simulink model "UnifiedPowerFlowController"  (R2024a)
settings: Solver=FixedStepDiscrete  StartTime=0.0  StopTime=0.8  FixedStep=Ts  RelTol=1e-3
PreLoadFcn:
  | Ts=1/512/60;
undefined symbols (not defined in the file or in its folder): DiscIntNeverNeededParam
libraries: spsabctodq0Lib x10, spsMeanVariableFrequencyLib x10, spsThreeLevelBridgeLib x8, spsVoltageMeasurementLib x8, spsZigzagPhaseShiftingTransformerLib x8, spsCurrentMeasurementLib x6, spsSecondOrderFilterLib x5, spsThreePhaseVIMeasurementLib x4, spsSeriesRLCBranchLib x4, spsDistributedParametersLineLib x3, spsPowerPositiveSequenceLib x3, spsThreePhaseSourceLib x2
(part 1 of 7)
settings Model: Creator=The MathWorks, Inc.  LastModifiedBy=Monia
settings SolverCC: AlgebraicLoopSolver=TrustRegion
settings DataIOCC: InitialState=xInitial_upfc  SaveFinalState=on  SaveFormat=Structure  SaveOutput=off  SaveTime=off  ReturnWorkspaceOutputs=off  SignalLoggingName=sigsOut
settings OptimizationCC: BlockReduction=off  BooleanDataType=off  ExpressionDepthLimit=2147483647  InitFltsAndDblsToZero=on  EfficientMapNaN2IntZero=off  LifeSpan=inf
settings DebuggingCC: UnderspecifiedInitializationDetection=Classic  MergeDetectMultiDrivingBlocksExec=none  SignalResolutionControl=TryResolveAllWithWarning  MultiTaskDSMMsg=warning  MultiTaskCondExecSysMsg=none  FcnCallInpInsideContextMsg=warning  UnconnectedInputMsg=warning  UnconnectedOutputMsg=warning  UnconnectedLineMsg=warning  StateNameClashWarn=warning  SFUnexpectedBacktrackingDiag=warning  SFNoUnconditionalDefaultTransitionDiag=warning  SFExecutionAtInitializationDiag=none  ArithmeticOperatorsInVariantConditions=warning
settings HardwareCC: ProdBitPerPointer=32  ProdBitPerSizeT=32  ProdBitPerPtrDiffT=32  ProdLargestAtomicFloat=None  ProdIntDivRoundTo=Undefined  ProdEndianess=Unspecified  ProdWordSize=32  ProdHWDeviceType=32-bit Generic  TargetBitPerPointer=64  TargetBitPerSizeT=64  TargetBitPerPtrDiffT=64  TargetLongLongMode=on  TargetIntDivRoundTo=Zero  TargetEndianess=LittleEndian  TargetWordSize=64  TargetHWDeviceType=MATLAB Host  ProdEqTarget=off
settings ModelReferenceCC: EnableRefExpFcnMdlSchedulingChecks=on  PropagateSignalLabelsOutOfModel=off
settings SFSimCC: SimUseLocalCustomCode=off  CustomCodeUndefinedFunction=UseInterfaceOnly
settings RTWCC: SystemTargetFile=accel.tlc  TemplateMakefile=accel_default_tmf  RTWUseLocalCustomCode=off  GPUComputeCapability=3.5  DLArmComputeVersion=19.05
settings CodeAppCC: StateflowObjectComments=on
settings STFCustomTargetCC: TargetLangStandard=C89/C90 (ANSI)  MATLABClassNameForMDSCustomization=Simulink.SoftwareTarget.TargetSpecificTriggerConfigurationBase  UseToolchainInfoCompliant=off  SystemTargetFile=accel.tlc
settings ConfigComp: CovMetricSettings=dw  CovSaveCumulativeToWorkspaceVar=on  CovSaveSingleToWorkspaceVar=on  CovExternalEMLEnable=off  CovSFcnEnable=off
settings SimscapeCC: SimscapeNormalizeSystem=off

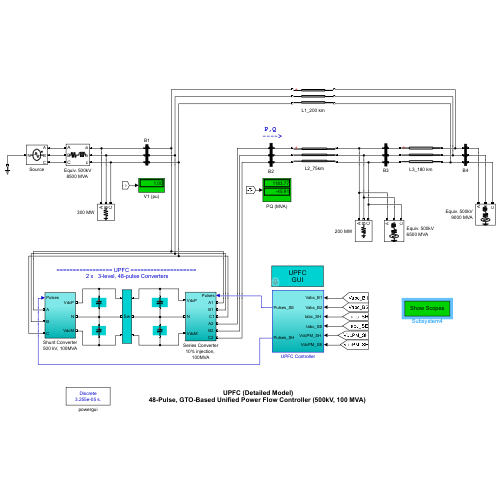
[thumbnail: Simulink's stored preview of the top-level diagram]
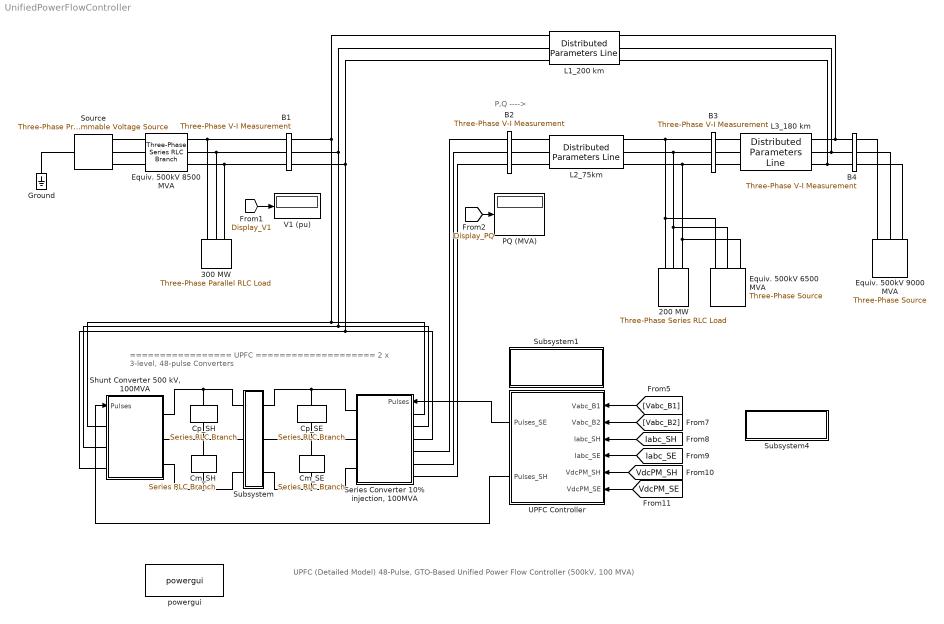
== system UnifiedPowerFlowController ==
  note: ================= UPFC ====================
      | 2 x   3-level, 48-pulse Converters
  note: P,Q
      | ---->
  note: UPFC (Detailed Model)
      | 48-Pulse, GTO-Based Unified Power Flow Controller (500kV, 100 MVA)
  200 MW : spsThreePhaseSeriesRLCLoadLib/Three-Phase Series RLC Load  LConnTagsString=A|B|C  Configuration=Y (grounded)  NominalVoltage=500e3  Vabc=[1e3 1e3 1e3]  Vabcp=[1e3 1e3 1e3]  NominalFrequency=60  UnbalancedPower=off  ActivePower=200e6  InductivePower=0  CapacitivePower=0  Pabc=[10e3 9e3 11e3]  QLabc=[100 90 110]  QCabc=[100 90 110]  Pabcp=[10e3 9e3 11e3]  QLabcp=[100 90 110]  QCabcp=[100 90 110]  Measurements=None  LoadType=constant Z
  300 MW : spsThreePhaseParallelRLCLoadLib/Three-Phase Parallel RLC Load  LConnTagsString=A|B|C  Configuration=Y (grounded)  NominalVoltage=500e3  Vabc=[1e3 1e3 1e3]  Vabcp=[1e3 1e3 1e3]  NominalFrequency=60  UnbalancedPower=off  ActivePower=300e6  InductivePower=0  CapacitivePower=0  Pabc=[10e3 9e3 11e3]  QLabc=[100 90 110]  QCabc=[100 90 110]  Pabcp=[10e3 9e3 11e3]  QLabcp=[100 90 110]  QCabcp=[100 90 110]  Measurements=None  LoadType=constant Z
  B1 : spsThreePhaseVIMeasurementLib/Three-Phase V-I Measurement  VoltageMeasurement=phase-to-ground  SetLabelV=on  LabelV=Vabc_B1  Vpu=on  VpuLL=off  CurrentMeasurement=yes  SetLabelI=on  LabelI=Iabc_B1  Ipu=on  Pbase=100e6  Vbase=500e3  OutputType=Magnitude  PhasorSimulation=off  PSBequivalent=0
  B2 : spsThreePhaseVIMeasurementLib/Three-Phase V-I Measurement  VoltageMeasurement=phase-to-ground  SetLabelV=on  LabelV=Vabc_B2  Vpu=on  VpuLL=off  CurrentMeasurement=yes  SetLabelI=on  LabelI=Iabc_B2  Ipu=on  Pbase=100e6  Vbase=500e3  OutputType=Magnitude  PhasorSimulation=off  PSBequivalent=0
  B3 : spsThreePhaseVIMeasurementLib/Three-Phase V-I Measurement  VoltageMeasurement=phase-to-ground  SetLabelV=on  LabelV=Vabc_B3  Vpu=on  VpuLL=off  CurrentMeasurement=yes  SetLabelI=on  LabelI=Iabc_B3  Ipu=on  Pbase=100e6  Vbase=500e3  OutputType=Magnitude  PhasorSimulation=off  PSBequivalent=0
  B4 : spsThreePhaseVIMeasurementLib/Three-Phase V-I Measurement  VoltageMeasurement=phase-to-ground  SetLabelV=on  LabelV=Vabc_B4  Vpu=on  VpuLL=off  CurrentMeasurement=no  SetLabelI=on  LabelI=Iabc_B4  Ipu=on  Pbase=100e6  Vbase=500e3  OutputType=Magnitude  PhasorSimulation=off  PSBequivalent=0
  Cm_SE : spsSeriesRLCBranchLib/Series RLC Branch  LConnTagsString=__new0  RConnTagsString=__new0  BranchType=C  Resistance=1.0  Inductance=1.0  SetiL0=off  InitialCurrent=0  Capacitance=2500e-6  Setx0=off  InitialVoltage=0  Measurements=Branch voltage
  Cm_SH : spsSeriesRLCBranchLib/Series RLC Branch  LConnTagsString=__new0  RConnTagsString=__new0  BranchType=C  Resistance=1.0  Inductance=1.0  SetiL0=off  InitialCurrent=0  Capacitance=2500e-6  Setx0=off  InitialVoltage=0  Measurements=Branch voltage
  Cp_SE : spsSeriesRLCBranchLib/Series RLC Branch  LConnTagsString=__new0  RConnTagsString=__new0  BranchType=C  Resistance=1.0  Inductance=1.0  SetiL0=off  InitialCurrent=0  Capacitance=2500e-6  Setx0=off  InitialVoltage=0  Measurements=Branch voltage
  Cp_SH : spsSeriesRLCBranchLib/Series RLC Branch  LConnTagsString=__new0  RConnTagsString=__new0  BranchType=C  Resistance=1.0  Inductance=1.0  SetiL0=off  InitialCurrent=0  Capacitance=2500e-6  Setx0=off  InitialVoltage=0  Measurements=Branch voltage
  Equiv. 500kV 6500 MVA : spsThreePhaseSourceLib/Three-Phase Source  InternalConnection=Yg  VoltagePhases=off  Voltage=500e3*1.00  PhaseAngle=9.2-20  Voltage_phases=[25e3 25e3 25e3]/sqrt(3)  PhaseAngles_phases=[0 -120 +120]  Frequency=60  NonIdealSource=on  SpecifyImpedance=on  Resistance=0.8929  Inductance=16.58e-3  ShortCircuitLevel=6500e6  BaseVoltage=500e3  XRratio=8  BusType=swing  Pref=0  Qref=0  Prefabc=[10e3, 10e3, 10e3]  Qrefabc=[0, 0, 0]  Qmin=-inf  Qmax=inf
  "Equiv. 500kV 8500 MVA " : spsThreePhaseSeriesRLCBranchLib/Three-Phase Series RLC Branch  LConnTagsString=A|B|C  RConnTagsString=A|B|C  BranchType=RL  Resistance=500e3^2/8500e6/10  Inductance=500e3^2/8500e6/(2*pi*60)  Capacitance=1.0  Measurements=None
  Equiv. 500kV 9000 MVA : spsThreePhaseSourceLib/Three-Phase Source  InternalConnection=Yg  VoltagePhases=off  Voltage=500e3*0.98  PhaseAngle=9.2-40  Voltage_phases=[25e3 25e3 25e3]/sqrt(3)  PhaseAngles_phases=[0 -120 +120]  Frequency=60  NonIdealSource=on  SpecifyImpedance=on  Resistance=0.8929  Inductance=16.58e-3  ShortCircuitLevel=9000e6  BaseVoltage=500e3  XRratio=10  BusType=swing  Pref=0  Qref=0  Prefabc=[10e3, 10e3, 10e3]  Qrefabc=[0, 0, 0]  Qmin=-inf  Qmax=inf
  Ground : spsGroundLib/Ground  LConnTagsString=a
  L1_200 km : spsDistributedParametersLineLib/Distributed Parameters Line  Phases=3  Length=200  Frequency=60  Resistance=[0.01273*2 0.3864]  Inductance="[0.9337e-3  4.1264e-3]"  Capacitance=[12.74e-9 7.751e-9]  x1=[-0.00113932291666667 -1.30080473974736e-10 4414.79498015263 -499890.552538387;-0.00110677083333333 -1.3001617192128e-10 10548.8886083546 -499798.73537353;-0.00107421875 -1.2993228991057e-10 16681.393612734 -499631.650357529;-0.00104166666666667 -1.29828840574929e-10 22811.3864605943 -499389.322652774;-0.00100911458333333 -1.29705839493444e-10 28937.9439975605 -499071.788752926;-0.0009765625 -1.29563305189627e-10 35060.1435866028 -498679.096477422;-0.000944010416666667 -1.2940125912862e-10 41177.0632469823 -498211.304964274;-0.000911458333333333 -1.29219725713964e-10 47287.7817930979 -497668.484661164;-0.00087890625 -1.29018732283922e-10 53391.3789732137 -497050.717314833;-0.000846354166666667 -1.28798309107367e-10 59486.935608045 -496358.09595877;-0.000813802083333333 -1.28558489379218e-10 65573.5337291838 -495590.724899204;-0.00078125 -1.28299309215443e-10 71650.2567173415 -494748.719699394;-0.000748697916666667 -1.28020807647623e-10 77716.1894403879 -493832.207162227;-0.000716145833333333 -1.27723026617068e-10 83770.4183911672 -492841.325311118;-0.00068359375 -1.27406010968507e-10 89812.0318250686 -491776.223369231;-0.000651041666666667 -1.2706980844333e-10 95840.1198973318 -490637.061736999;-0.000618489583333333 -1.26714469672401e-10 101853.774800066 -489424.011967975;-0.0005859375 -1.26340048168432e-10 107852.090898963 -488137.256742991;-0.000553385416666667 -1.25946600317924e-10 113834.164869682 -486776.989842652;-0.000520833333333333 -1.25534185372677e-10 119799.095833886 -485343.416118148;-0.00048828125 -1.25102865440863e-10 125745.985494914 -483836.751460411;-0.000455729166666667 -1.24652705477678e-10 131673.938273056 -482257.222767596;-0.000423177083333333 -1.24183773275557e-10 137582.061440429 -480605.067910913;-0.000390625 -1.23696139453964e-10 143469.465255415 -478880.535698807;-0.000358072916666667 -1.2318987744876e-10 149335.263096657 -477083.885839486;-0.000325520833333333 -1.2266506350114e-10 155178.571596574 -475215.388901809;-0.00029296875 -1.22121776646154e-10 160998.5107744 -473275.326274544;-0.000260416666666667 -1.21560098700805e-10 166794.204168703 -471263.990123985;-0.000227864583333333 -1.20980114251724e-10 172564.778969376 -469181.683349959;-0.0001953125 -1.20381910642437e-10 178309.366149078 -467028.719540206;-0.000162760416666667 -1.19765577960207e-10 184027.100594112 -464805.422923158;-0.000130208333333333 -1.19131209022468e-10 189717.121234702 -462512.128319105;-9.765625e-05 -1.1847889936285e-10 195378.571174668 -460149.181089781;-6.51041666666667e-05 -1.17808747216787e-10 201010.597820474 -457716.937086347;-3.25520833333333e-05 -1.17120853506728e-10 206612.353009623 -455215.762595802]  x2=[-0.00113932291666667 -1.05841083346228e-10 -126400.807658291 -476001.468702008;-0.00110677083333333 -1.0642802292755e-10 -120550.019662708 -477516.759017374;-0.00107421875 -1.06998934840092e-10 -114681.077277581 -478960.137065278;-0.00104166666666667 -1.0755373310662e-10 -108794.864344047 -480331.385478293;-0.00100911458333333 -1.08092334176555e-10 -102892.267304122 -481630.297751453;-0.0009765625 -1.08614656938559e-10 -96974.175067208 -482856.678273347;-0.000944010416666667 -1.09120622732743e-10 -91041.4788762281 -484010.34235558;-0.000911458333333333 -1.09610155362522e-10 -85095.0721734062 -485091.116260584;-0.00087890625 -1.1008318110608e-10 -79135.8504657194 -486098.837227784;-0.000846354166666667 -1.10539628727482e-10 -73164.7111900368 -487033.35349811;-0.000813802083333333 -1.10979429487394e-10 -67182.5535779701 -487894.524336849;-0.00078125 -1.1140251715344e-10 -61190.2785204513 -488682.220054839;-0.000748697916666667 -1.11808828010173e-10 -55188.7884320629 -489396.322028004;-0.000716145833333333 -1.12198300868673e-10 -49178.987115137 -490036.722715212;-0.00068359375 -1.1257087707576e-10 -43161.7796236461 -490603.325674476;-0.000651041666666667 -1.12926500522828e-10 -37138.0721269053 -491096.045577475;-0.000618489583333333 -1.13265117654293e-10 -31108.7717731068 -491514.808222403;-0.0005859375 -1.13586677475661e-10 -25074.7865527063 -491859.550545146;-0.000553385416666667 -1.13891131561206e-10 -19037.0251616833 -492130.220628778;-0.000520833333333333 -1.14178434061263e-10 -12996.3968646946 -492326.777711381;-0.00048828125 -1.14448541709131e-10 -6953.8113581426 -492449.192192181;-0.000455729166666667 -1.14701413827592e-10 -910.178633178191 -492497.445636008;-0.000423177083333333 -1.14937012335036e-10 5133.59116134048 -492471.530776069;-0.000390625 -1.15155301751194e-10 11176.5878559131 -492371.451515048;-0.000358072916666667 -1.15356249202483e-10 17217.9013974653 -492197.222924514;-0.000325520833333333 -1.15539824426955e-10 23256.6219863995 -491948.871242651;-0.00029296875 -1.15705999778858e-10 29291.8402136071 -491626.433870309;-0.000260416666666667 -1.15854750232794e-10 35322.6471974224 -491229.95936537;-0.000227864583333333 -1.15986053387492e-10 41348.1347204966 -490759.507435436;-0.0001953125 -1.16099889469181e-10 47367.3953665724 -490215.148928839;-0.000162760416666667 -1.16196241334564e-10 53379.5226571369 -489596.965823965;-0.000130208333333333 -1.16275094473405e-10 59383.6111879346 -488905.051216918;-9.765625e-05 -1.16336437010713e-10 65378.7567653174 -488139.509307491;-6.51041666666667e-05 -1.16380259708525e-10 71364.0565424134 -487300.455383481;-3.25520833333333e-05 -1.16406555967306e-10 77338.6091550917 -486388.015803322]  x3=[-0.00113932291666667 -2.8339490666223e-13 -16.9421274649165 53.6415754395801;-0.00110677083333333 -2.86603709471157e-13 -17.5991164005906 53.4296303617768;-0.00107421875 -2.89769350815649e-13 -18.2534549740693 53.2096389781707;-0.00104166666666667 -2.92891353961764e-13 -18.9050446443705 52.9816344186548;-0.00100911458333333 -2.95969248747311e-13 -19.5537872844865 52.7456510198773;-0.0009765625 -2.99002571652657e-13 -20.1995851961618 52.50172432007;-0.000944010416666667 -3.0199086587053e-13 -20.8423411246066 52.2498910536966;-0.000911458333333333 -3.04933681374813e-13 -21.4819582731421 51.9901891459206;-0.00087890625 -3.07830574988315e-13 -22.1183403177786 51.7226577068943;-0.000846354166666667 -3.10681110449514e-13 -22.7513914217208 51.4473370258682;-0.000813802083333333 -3.13484858478254e-13 -23.3810162498012 51.1642685651241;-0.00078125 -3.16241396840395e-13 -24.0071199828364 50.8734949537312;-0.000748697916666667 -3.18950310411399e-13 -24.6296083319074 50.5750599811256;-0.000716145833333333 -3.21611191238846e-13 -25.2483875525584 50.2690085905165;-0.00068359375 -3.24223638603872e-13 -25.8633644589148 49.9553868721177;-0.000651041666666667 -3.26787259081513e-13 -26.4744464377167 49.6342420562063;-0.000618489583333333 -3.29301666599954e-13 -27.0815414622657 49.3056225060103;-0.0005859375 -3.31766482498671e-13 -27.6845581062843 48.9695777104252;-0.000553385416666667 -3.34181335585458e-13 -28.2834055576838 48.6261582765612;-0.000520833333333333 -3.3654586219232e-13 -28.8779936322409 48.2754159221218;-0.00048828125 -3.3885970623025e-13 -29.4682327871786 47.9174034676155;-0.000455729166666667 -3.41122519242845e-13 -30.0540341346512 47.552174828401;-0.000423177083333333 -3.43333960458789e-13 -30.6353094551306 47.179785006568;-0.000390625 -3.4549369684317e-13 -31.2119712106915 46.800290082654;-0.000358072916666667 -3.47601403147632e-13 -31.7839325581948 46.4137472071984;-0.000325520833333333 -3.49656761959359e-13 -32.3511073623653 46.0202145921366;-0.00029296875 -3.51659463748873e-13 -32.9134102087637 45.619751502033;-0.000260416666666667 -3.53609206916652e-13 -33.4707564166498 45.2124182451557;-0.000227864583333333 -3.55505697838545e-13 -34.0230620517346 44.7982761643951;-0.0001953125 -3.57348650909997e-13 -34.5702439388211 44.3773876280251;-0.000162760416666667 -3.59137788589054e-13 -35.1122196743297 43.9498160203112;-0.000130208333333333 -3.60872841438162e-13 -35.6489076387083 43.5156257319647;-9.765625e-05 -3.62553548164744e-13 -36.1802270087235 43.0748821504461;-6.51041666666667e-05 -3.64179655660549e-13 -36.7060977696325 42.6276516501175;-3.25520833333333e-05 -3.65750919039769e-13 -37.226440727233 42.1740015822472]  x4=[-0.00113932291666667 -5.53609918313425e-14 -894.269601115783 -3549.34214309645;-0.00110677083333333 -6.65829424292671e-14 -850.646376261383 -3560.04894780867;-0.00107421875 -7.77948658809732e-14 -806.895047191641 -3570.21962224425;-0.00104166666666667 -8.89950737120296e-14 -763.022202695785 -3579.85263473701;-0.00100911458333333 -1.00181879212335e-13 -719.034449862819 -3588.94653459072;-0.0009765625 -1.11353597690128e-13 -674.938413086521 -3597.4999522975;-0.000944010416666667 -1.225085467257e-13 -630.740733067831 -3605.51159974411;-0.000911458333333333 -1.33645046424757e-13 -586.448065814787 -3612.98027040591;-0.00087890625 -1.44761419671408e-13 -542.067081640157 -3619.90483952857;-0.000846354166666667 -1.5585599238073e-13 -497.604464156912 -3626.28426429746;-0.000813802083333333 -1.66927093750883e-13 -453.066909271697 -3632.11758399467;-0.00078125 -1.77973056514724e-13 -408.461124176457 -3637.4039201437;-0.000748697916666667 -1.8899221719089e-13 -363.793826338355 -3642.14247664178;-0.000716145833333333 -1.99982916334315e-13 -319.071742488145 -3646.33253987974;-0.00068359375 -2.10943498786134e-13 -274.301607607154 -3649.97347884945;-0.000651041666666667 -2.21872313922948e-13 -229.490163913017 -3653.06474523891;-0.000618489583333333 -2.32767715905396e-13 -184.644159844327 -3655.60587351476;-0.0005859375 -2.43628063926015e-13 -139.770349044339 -3657.59648099244;-0.000553385416666667 -2.54451722456341e-13 -94.8754893439008 -3659.03626789378;-0.000520833333333333 -2.65237061493213e-13 -49.9663417437466 -3659.92501739216;-0.00048828125 -2.75982456804242e-13 -5.04966939631674 -3660.26259564519;-0.000455729166666667 -2.86686290172419e-13 39.8677634127503 -3660.04895181481;-0.000423177083333333 -2.97346949639812e-13 84.7791922832927 -3659.28411807502;-0.000390625 -3.07962829750317e-13 129.677853719319 -3657.96820960694;-0.000358072916666667 -3.18532331791438e-13 174.556986147569 -3656.10142458156;-0.000325520833333333 -3.29053864035045e-13 219.409830935775 -3653.68404412984;-0.00029296875 -3.39525841977084e-13 264.229633410495 -3650.71643230038;-0.000260416666666667 -3.49946688576195e-13 309.009643874337 -3647.1990360046;-0.000227864583333333 -3.60314834491212e-13 353.743118622438 -3643.13238494946;-0.0001953125 -3.70628718317496e-13 398.423320958044 -3638.51709155763;-0.000162760416666667 -3.80886786822081e-13 443.043522207029 -3633.35385087534;-0.000130208333333333 -3.91087495177583e-13 487.597002731213 -3627.64344046763;-9.765625e-05 -4.01229307194844e-13 532.077052940308 -3621.3867203013;-6.51041666666667e-05 -4.11310695554278e-13 576.476974302363 -3614.58463261541;-3.25520833333333e-05 -4.21330142035882e-13 620.790080352538 -3607.23820177933]  x5=0.00113108313399148  V1=ones(3,3)  V2=ones(3,3)  I1=ones(3,3)  I2=ones(3,3)  nHarmo=1  Measurements=None  Decoupling=off  VsMag0=0  VrMag0=0  VsAngle0=0  VrAngle0=0  IsMag0=0  IrMag0=0  IsAngle0=0  IrAngle0=0
      settings: AttributesFormatString=\n
  L2_75km : spsDistributedParametersLineLib/Distributed Parameters Line  Phases=3  Length=75  Frequency=60  Resistance=[0.01273*2 0.3864]  Inductance="[0.9337e-3  4.1264e-3]"  Capacitance=[12.74e-9 7.751e-9]  x1=[-0.000455729166666667 -2.0819094293585e-10 0 0;-0.000423177083333333 -2.08074842291704e-10 0 0;-0.000390625 -2.07927406341667e-10 0 0;-0.000358072916666667 -2.07748657289053e-10 0 0;-0.000325520833333333 -2.0753862205281e-10 0 0;-0.00029296875 -2.07297332263474e-10 0 0;-0.000260416666666667 -2.07024824258398e-10 166794.132131736 -471263.82102114;-0.000227864583333333 -2.06721139076285e-10 172564.704862681 -469181.515143851;-0.0001953125 -2.06386322451008e-10 178309.289983816 -467028.552256167;-0.000162760416666667 -2.06020424804719e-10 184027.022381753 -464805.256586379;-0.000130208333333333 -2.05623501240256e-10 189717.040987023 -462511.962954637;-9.765625e-05 -2.0519561153285e-10 195378.488903755 -460149.016722528;-6.51041666666667e-05 -2.04736820121115e-10 201010.513538717 -457716.77374106;-3.25520833333333e-05 -2.04247196097352e-10 206612.266729715 -455215.600297082]  x2=[-0.000455729166666667 1.24391145626069e-11 0 0;-0.000423177083333333 1.15584511756505e-11 0 0;-0.000390625 1.06760471284624e-11 0 0;-0.000358072916666667 9.79203530784625e-12 0 0;-0.000325520833333333 8.90654884273071e-12 0 0;-0.00029296875 8.01972108412033e-12 0 0;-0.000260416666666667 7.13168558501352e-12 120220.444766576 -484737.668130302;-0.000227864583333333 6.24257608029001e-12 126159.86924118 -483225.878484715;-0.0001953125 5.35252646657081e-12 132080.294503528 -481641.316799273;-0.000162760416666667 4.46167078205388e-12 137980.828959354 -479984.221703137;-0.000130208333333333 3.5701431863285e-12 143860.584009871 -478254.842748733;-9.765625e-05 2.67807794017127e-12 149718.674185598 -476453.440374171;-6.51041666666667e-05 1.78560938532699e-12 155554.2172797 -474580.285864021;-3.25520833333333e-05 8.92871924277273e-13 161366.334480854 -472635.661308464]  x3=[-0.000455729166666667 -2.11066122635043e-13 0 0;-0.000423177083333333 -1.95623086927928e-13 0 0;-0.000390625 -1.80150591103479e-13 0 0;-0.000358072916666667 -1.64650965262656e-13 0 0;-0.000325520833333333 -1.49126543592098e-13 0 0;-0.00029296875 -1.33579664012606e-13 0 0;-0.000260416666666667 -1.18012667827058e-13 -104.968306035296 -46.5279101834563;-0.000227864583333333 -1.0242789936782e-13 -104.389433083733 -47.8125293036903;-0.0001953125 -8.68277056436964e-14 -103.794839467522 -49.0899480328796;-0.000162760416666667 -7.12144359864806e-14 -103.184614730274 -50.3599739964621;-0.000130208333333333 -5.55904416971524e-14 -102.558850769591 -51.6224159331993;-9.765625e-05 -3.99580756917824e-14 -101.917641823223 -52.8770837239791;-6.51041666666667e-05 -2.43196921471906e-14 -101.261084454879 -54.1237884204473;-3.25520833333333e-05 -8.6776461464162e-15 -100.589277539683 -55.3623422734623]  x4=[-0.000455729166666667 -7.46107992302532e-13 0 0;-0.000423177083333333 -7.89283969106343e-13 0 0;-0.000390625 -8.32341082647621e-13 0 0;-0.000358072916666667 -8.75272848683443e-13 0 0;-0.000325520833333333 -9.1807280184776e-13 0 0;-0.00029296875 -9.60734496625056e-13 0 0;-0.000260416666666667 -1.00325150832102e-12 987.851977766536 -3517.72393741717;-0.000227864583333333 -1.04561743403008e-12 1030.94547830602 -3505.3365959085;-0.0001953125 -1.08782589359966e-12 1073.88372224859 -3492.42136360213;-0.000162760416666667 -1.129870530591e-12 1116.66024325264 -3478.98018548453;-0.000130208333333333 -1.17174501323642e-12 1159.26859933146 -3465.0150857477;-9.765625e-05 -1.21344303539287e-12 1201.70237382334 -3450.52816748428;-6.51041666666667e-05 -1.25495831749158e-12 1243.95517635793 -3435.52161237087;-3.25520833333333e-05 -1.29628460748377e-12 1286.0206438186 -3419.99768033948]  x5=0.000424156175246807  V1=ones(3,3)  V2=ones(3,3)  I1=ones(3,3)  I2=ones(3,3)  nHarmo=1  Measurements=None  Decoupling=off  VsMag0=0  VrMag0=0  VsAngle0=0  VrAngle0=0  IsMag0=0  IrMag0=0  IsAngle0=0  IrAngle0=0
      settings: AttributesFormatString=\n
  L3_180 km : spsDistributedParametersLineLib/Distributed Parameters Line  Phases=3  Length=180  Frequency=60  Resistance=[0.01273*2 0.3864]  Inductance="[0.9337e-3  4.1264e-3]"  Capacitance=[12.74e-9 7.751e-9]  x1=[-0.00104166666666667 2.78438843353862e-11 0 0;-0.00100911458333333 2.7016881646111e-11 0 0;-0.0009765625 2.61858103138357e-11 0 0;-0.000944010416666667 2.53507954948461e-11 0 0;-0.000911458333333333 2.45119629393026e-11 0 0;-0.00087890625 2.36694389723025e-11 0 0;-0.000846354166666667 2.28233504748562e-11 0 0;-0.000813802083333333 2.19738248647793e-11 0 0;-0.00078125 2.11209900775038e-11 0 0;-0.000748697916666667 2.02649745468118e-11 0 0;-0.000716145833333333 1.94059071854934e-11 0 0;-0.00068359375 1.85439173659335e-11 0 0;-0.000651041666666667 1.76791349006281e-11 47793.4519494709 -497131.117709433;-0.000618489583333333 1.68116900226357e-11 53890.4167344322 -496507.185475161;-0.0005859375 1.59417133659641e-11 59979.2658208579 -495808.481085053;-0.000553385416666667 1.50693359458978e-11 66059.0822504719 -495035.109761421;-0.000520833333333333 1.41946891392674e-11 72128.9504252835 -494187.18797114;-0.00048828125 1.33179046646649e-11 78187.9562454721 -493264.843408115;-0.000455729166666667 1.24391145626069e-11 84235.1872470482 -492268.214974043;-0.000423177083333333 1.15584511756505e-11 90269.7327392661 -491197.452757501;-0.000390625 1.06760471284624e-11 96290.6839417718 -490052.71801134;-0.000358072916666667 9.79203530784625e-12 102297.134121461 -488834.183128402;-0.000325520833333333 8.90654884273071e-12 108288.178729029 -487542.031615558;-0.00029296875 8.01972108412032e-12 114262.915535197 -486176.458066074;-0.000260416666666667 7.13168558501352e-12 120220.444766576 -484737.668130302;-0.000227864583333333 6.24257608029001e-12 126159.86924118 -483225.878484715;-0.0001953125 5.35252646657081e-12 132080.294503528 -481641.316799273;-0.000162760416666667 4.46167078205388e-12 137980.828959354 -479984.221703137;-0.000130208333333333 3.5701431863285e-12 143860.584009871 -478254.842748733;-9.765625e-05 2.67807794017127e-12 149718.674185598 -476453.440374171;-6.51041666666667e-05 1.78560938532699e-12 155554.2172797 -474580.285864021;-3.25520833333333e-05 8.92871924277273e-13 161366.334480854 -472635.661308464]  x2=[-0.00104166666666667 -8.06652998299646e-11 0 0;-0.00100911458333333 -8.10692506324164e-11 0 0;-0.0009765625 -8.14609927039191e-11 0 0;-0.000944010416666667 -8.18404670495576e-11 0 0;-0.000911458333333333 -8.22076165218914e-11 0 0;-0.00087890625 -8.25623858295603e-11 0 0;-0.000846354166666667 -8.29047215456117e-11 0 0;-0.000813802083333333 -8.32345721155458e-11 0 0;-0.00078125 -8.35518878650801e-11 0 0;-0.000748697916666667 -8.38566210076299e-11 0 0;-0.000716145833333333 -8.41487256515049e-11 0 0;-0.00068359375 -8.44281578068201e-11 0 0;-0.000651041666666667 -8.46948753921208e-11 -37138.0721269053 -491096.045577475;-0.000618489583333333 -8.49488382407197e-11 -31108.7717731068 -491514.808222403;-0.0005859375 -8.51900081067458e-11 -25074.7865527063 -491859.550545146;-0.000553385416666667 -8.54183486709046e-11 -19037.0251616833 -492130.220628778;-0.000520833333333333 -8.56338255459469e-11 -12996.3968646946 -492326.777711381;-0.00048828125 -8.5836406281848e-11 -6953.8113581426 -492449.192192181;-0.000455729166666667 -8.60260603706941e-11 -910.178633178191 -492497.445636008;-0.000423177083333333 -8.62027592512772e-11 5133.59116134048 -492471.530776069;-0.000390625 -8.63664763133956e-11 11176.5878559131 -492371.451515048;-0.000358072916666667 -8.65171869018622e-11 17217.9013974653 -492197.222924514;-0.000325520833333333 -8.66548683202165e-11 23256.6219863995 -491948.871242651;-0.00029296875 -8.67794998341434e-11 29291.8402136071 -491626.433870309;-0.000260416666666667 -8.68910626745955e-11 35322.6471974224 -491229.95936537;-0.000227864583333333 -8.69895400406192e-11 41348.1347204966 -490759.507435436;-0.0001953125 -8.70749171018854e-11 47367.3953665724 -490215.148928839;-0.000162760416666667 -8.71471810009228e-11 53379.5226571369 -489596.965823965;-0.000130208333333333 -8.7206320855054e-11 59383.6111879346 -488905.051216918;-9.765625e-05 -8.72523277580345e-11 65378.7567653174 -488139.509307491;-6.51041666666667e-05 -8.72851947813939e-11 71364.0565424134 -487300.455383481;-3.25520833333333e-05 -8.73049169754794e-11 77338.6091550917 -486388.015803322]  x3=[-0.00104166666666667 8.73001351836037e-13 0 0;-0.00100911458333333 8.70534247994934e-13 0 0;-0.0009765625 8.6793604489816e-13 0 0;-0.000944010416666667 8.65207133825544e-13 0 0;-0.000911458333333333 8.62347925741056e-13 0 0;-0.00087890625 8.59358851230916e-13 0 0;-0.000846354166666667 8.56240360438751e-13 0 0;-0.000813802083333333 8.52992922997804e-13 0 0;-0.00078125 8.49617027960207e-13 0 0;-0.000748697916666667 8.46113183723337e-13 0 0;-0.000716145833333333 8.42481917953247e-13 0 0;-0.00068359375 8.38723777505205e-13 0 0;-0.000651041666666667 8.3483932834134e-13 -40.336635661739 -492.384145706459;-0.000618489583333333 8.30829155445406e-13 -34.2912874919403 -492.842062654693;-0.0005859375 8.26693862734693e-13 -28.2407751803785 -493.225759401107;-0.000553385416666667 8.2243407296907e-13 -22.1860099119524 -493.535178162382;-0.000520833333333333 8.18050427657209e-13 -16.12790351204 -493.770272341191;-0.00048828125 8.13543586959969e-13 -10.0673683091819 -493.931006533215;-0.000455729166666667 8.0891422959098e-13 -4.00531699768707 -494.017356532476;-0.000423177083333333 8.04163052714436e-13 2.05733749981491 -494.029309334982;-0.000390625 7.99290771840097e-13 8.11968216985689 -493.966863140685;-0.000358072916666667 7.94298120715542e-13 14.1808040456306 -493.830027353751;-0.000325520833333333 7.89185851215665e-13 20.2397903444762 -493.618822581148;-0.00029296875 7.83954733229448e-13 26.2957286053437 -493.333280629537;-0.000260416666666667 7.7860555454402e-13 32.3477068262065 -492.973444500485;-0.000227864583333333 7.73139120726013e-13 38.3948136014055 -492.539368383991;-0.0001953125 7.67556255000254e-13 44.4361382589033 -492.03111765032;-0.000162760416666667 7.61857798125786e-13 50.4707709974284 -491.448768840164;-0.000130208333333333 7.56044608269253e-13 56.4978030234873 -490.79240965311;-9.765625e-05 7.50117560875666e-13 62.5163266882261 -490.06213893444;-6.51041666666667e-05 7.4407754853656e-13 68.5254356241187 -489.258066660236;-3.25520833333333e-05 7.37925480855577e-13 74.5242248814628 -488.380313920826]  x4=[-0.00104166666666667 -1.03966132158043e-12 0 0;-0.00100911458333333 -1.03658904593954e-12 0 0;-0.0009765625 -1.0333606638012e-12 0 0;-0.000944010416666667 -1.02997666134789e-12 0 0;-0.000911458333333333 -1.02643754819794e-12 0 0;-0.00087890625 -1.02274385732876e-12 0 0;-0.000846354166666667 -1.01889614499662e-12 0 0;-0.000813802083333333 -1.01489499065283e-12 0 0;-0.00078125 -1.01074099685653e-12 0 0;-0.000748697916666667 -1.00643478918389e-12 0 0;-0.000716145833333333 -1.00197701613397e-12 0 0;-0.00068359375 -9.97368349030976e-13 0 0;-0.000651041666666667 -9.92609481923228e-13 -346.315027735525 -3116.34913325067;-0.000618489583333333 -9.87701131478607e-13 -308.046553150504 -3120.36429601412;-0.0005859375 -9.82644036876635e-13 -269.731687887663 -3123.90954339221;-0.000553385416666667 -9.77438959697159e-13 -231.376202024778 -3126.9843414837;-0.000520833333333333 -9.72086683805655e-13 -192.985871756935 -3129.58822723531;-0.00048828125 -9.66588015235186e-13 -154.566478526665 -3131.72080851143;-0.000455729166666667 -9.60943782065013e-13 -116.123808153268 -3133.38176415317;-0.000423177083333333 -9.5515483429589e-13 -77.6636499615 -3134.5708440267;-0.000390625 -9.49222043722057e-13 -39.1917959097174 -3135.28786906099;-0.000358072916666667 -9.43146303799953e-13 -0.714039717629646 -3135.53273127469;-0.000325520833333333 -9.36928529513661e-13 37.7638240062132 -3135.30539379245;-0.00029296875 -9.30569657237119e-13 76.236000637067 -3134.60589085047;-0.000260416666666667 -9.24070644593101e-13 114.696696406643 -3133.43432779132;-0.000227864583333333 -9.17432470309006e-13 153.140119275627 -3131.79088104807;-0.0001953125 -9.10656134069465e-13 191.560479805943 -3129.67579811778;-0.000162760416666667 -9.03742656365789e-13 229.951992032614 -3127.08939752414;-0.000130208333333333 -8.96693078342291e-13 268.308874335115 -3124.03206876957;-9.765625e-05 -8.89508461639491e-13 306.625350308059 -3120.50427227653;-6.51041666666667e-05 -8.82189888234238e-13 344.895649631104 -3116.50653931821;-3.25520833333333e-05 -8.74738460276766e-13 383.114008937939 -3112.03947193848]  x5=0.00101797482059234  V1=ones(3,3)  V2=ones(3,3)  I1=ones(3,3)  I2=ones(3,3)  nHarmo=1  Measurements=None  Decoupling=off  VsMag0=0  VrMag0=0  VsAngle0=0  VrAngle0=0  IsMag0=0  IrMag0=0  IsAngle0=0  IrAngle0=0
      settings: AttributesFormatString=\n
  PQ (MVA) : Display
      settings: Format=bank  SampleTime=Ts*100
  "Series Converter 10% injection, 100MVA" : Subsystem
  "Shunt Converter 500 kV, 100MVA" : Subsystem
  Source : spsThreePhaseProgrammableVoltageSourceLib/Three-Phase Programmable Voltage Source  PositiveSequence="[500e3*1.0491 9.2  60]"  VariationEntity=None  VariationType=Modulation  VariationTypeAlt=Step  VariationStep=-0.3  VariationRate=0.5  VariationMagnitude=0.4  VariationFrequency=2  VariationTiming=[0.1 1.2]  VariationPhaseA=off  Amplitudes="[1  0.8  1.2  1.0 ]"  TimeValues=[0 0.1 0.25 0.4]  HarmonicGeneration=off  HarmonicA=[3 0.2 -25 0]  HarmonicB="[2 0.15  35 2]"  Timing="[0.1  0.6]"  BusType=swing  Pref=0  Qref=0  Qmin=-inf  Qmax=inf
  Subsystem : Subsystem
      mask Display: disp('Sw')
  Subsystem1 : Subsystem  mask(UPFC GUI){OpMode=SSSC (Voltage Injection), Par_VarControl=[0.3  0.5  +0.8  -0.8 ], Par_Vref=[ 1  1.005  0.3 *100], Par_SSSC=[ 0.0  0.08  0.3  ], Par_UPFC_Pref=[  +8.7  +10   0.25  ], Par_UPFC_Qref=[  -0.6  +0.7  0.5  ]}
      mask prompts: OpMode "Operation Mode:"; Par_VarControl "STATCOM (Qref): [T1 T2 Q1 Q2]"; Par_Vref "STATCOM Vref (pu): [ Initial   Final  StepTime ]"; Par_SSSC "SSSC Votage Injection (pu): [ Initial  Final  StepTime ]"; Par_UPFC_Pref "UPFC Pref (pu): [ Initial  Final  StepTime ]"; Par_UPFC_Qref "UPFC Qref (pu): [ Initial  Final  StepTime ]"
      mask TypeOptions OpMode: STATCOM (Var Control) | STATCOM (Voltage Control) | SSSC (Voltage Injection) | STATCOM  (Voltage Control) + SSSC (Voltage Injection) | UPFC  (Power Flow Control)
      mask Display: disp('UPFC\nGUI')
  Subsystem4 : Subsystem
      mask Display: disp('Show Scopes')
  UPFC Controller : Subsystem
  V1 (pu) : Display
      settings: Format=bank  SampleTime=Ts*100
  powergui : spspowerguiLib/powergui  Priority=2  SimulationMode=Discrete  SampleTime=Ts  frequency=60  Iterations=50  frequencyindice=60  Pbase=100e6  ErrMax=1e-4  UnitsV=kV  UnitsW=MW  buscounter=0  FunctionMessages=off  echomessages=off  EnableUseOfTLC=off  CurrentSourceSwitches=off  DisableSnubberDevices=off  DisableRonSwitches=off  DisableVfSwitches=off  DisplayEquations=off  AutomaticDiscreteSolvers=off  SolverType=Tustin/Backward Euler (TBE)  Interpol=off  ExternalGateDelay=off  methode=off  Ts=0  x0status=blocks  SPID=off  SwTol=0  HookPort=off  NonlinearTolerance=1e-4  nMaxIteration=100  ContinueOnMaxIteration=off  RestoreLinks=yes  ResistiveCurrentMeasurement=off  Frange=[0:2:500]  Ylog=off  Xlog=on  ShowGrid=off  save=off  variable=ZData  structure=0  ZoomFFT=on  StartTime=0.0  cycles=1  DisplayStyle=1  fundamental=60  FreqAxis=off  MaxFrequency=1000  frequencyindicesteady=1  RmsSteady=1  display=off
  wires:
  [Vabc_B1] -> UPFC Controller/1(Vabc_B1)
  [Vabc_B2] -> UPFC Controller/2(Vabc_B2)
  [Iabc_SH] -> UPFC Controller/3("Iabc_SH ")
  [Iabc_SE] -> UPFC Controller/4(Iabc_SE)
  [VdcPM_SH] -> UPFC Controller/5("VdcPM_SH ")
  [VdcPM_SE] -> UPFC Controller/6(VdcPM_SE)
  [Display_V1] -> V1 (pu)/1
  [Display_PQ] -> PQ (MVA)/1
  UPFC Controller/2(Pulses_SH) -> "Shunt Converter 500 kV, 100MVA"/1(Pulses)
  UPFC Controller/1(Pulses_SE) -> "Series Converter 10% injection, 100MVA"/1(Pulses)
  connections:
  Ground/LConn1 -- Source/LConn1
  Source/RConn1 -- "Equiv. 500kV 8500 MVA "/LConn1
  Source/RConn2 -- "Equiv. 500kV 8500 MVA "/LConn2
  Source/RConn3 -- "Equiv. 500kV 8500 MVA "/LConn3
  Subsystem/LConn2 -- "Shunt Converter 500 kV, 100MVA"/RConn2 -- Cp_SH/RConn1 -- Cm_SH/LConn1
  Subsystem/RConn3 -- "Series Converter 10% injection, 100MVA"/RConn3 -- Cm_SE/RConn1
  Subsystem/RConn1 -- "Series Converter 10% injection, 100MVA"/RConn1 -- Cp_SE/LConn1
  B3/LConn1 -- 200 MW/LConn1 -- Equiv. 500kV 6500 MVA/RConn1 -- L2_75km/RConn1
  B3/LConn2 -- 200 MW/LConn2 -- Equiv. 500kV 6500 MVA/RConn2 -- L2_75km/RConn2
  B3/LConn3 -- 200 MW/LConn3 -- Equiv. 500kV 6500 MVA/RConn3 -- L2_75km/RConn3
  "Equiv. 500kV 8500 MVA "/RConn2 -- 300 MW/LConn2 -- B1/LConn2
  "Equiv. 500kV 8500 MVA "/RConn3 -- 300 MW/LConn3 -- B1/LConn3
  B2/RConn1 -- L2_75km/LConn1
  B2/RConn2 -- L2_75km/LConn2
  B2/RConn3 -- L2_75km/LConn3
  B3/RConn1 -- L3_180 km/LConn1
  B3/RConn2 -- L3_180 km/LConn2
  B3/RConn3 -- L3_180 km/LConn3
  300 MW/LConn1 -- "Equiv. 500kV 8500 MVA "/RConn1 -- B1/LConn1
  L3_180 km/RConn1 -- B4/LConn1 -- L1_200 km/RConn1
  L3_180 km/RConn2 -- B4/LConn2 -- L1_200 km/RConn2
  L3_180 km/RConn3 -- B4/LConn3 -- L1_200 km/RConn3
  B4/RConn1 -- Equiv. 500kV 9000 MVA/RConn1
  B4/RConn2 -- Equiv. 500kV 9000 MVA/RConn2
  B4/RConn3 -- Equiv. 500kV 9000 MVA/RConn3
  "Shunt Converter 500 kV, 100MVA"/LConn1 -- "Series Converter 10% injection, 100MVA"/LConn1 -- L1_200 km/LConn1 -- B1/RConn1
  B1/RConn2 -- L1_200 km/LConn2 -- "Series Converter 10% injection, 100MVA"/LConn2 -- "Shunt Converter 500 kV, 100MVA"/LConn2
  "Shunt Converter 500 kV, 100MVA"/LConn3 -- "Series Converter 10% injection, 100MVA"/LConn3 -- L1_200 km/LConn3 -- B1/RConn3
  "Series Converter 10% injection, 100MVA"/LConn4 -- B2/LConn1
  B2/LConn2 -- "Series Converter 10% injection, 100MVA"/LConn5
  B2/LConn3 -- "Series Converter 10% injection, 100MVA"/LConn6
  Subsystem/RConn2 -- "Series Converter 10% injection, 100MVA"/RConn2 -- Cm_SE/LConn1 -- Cp_SE/RConn1
  "Shunt Converter 500 kV, 100MVA"/RConn1 -- Subsystem/LConn1 -- Cp_SH/LConn1
  "Shunt Converter 500 kV, 100MVA"/RConn3 -- Subsystem/LConn3 -- Cm_SH/RConn1

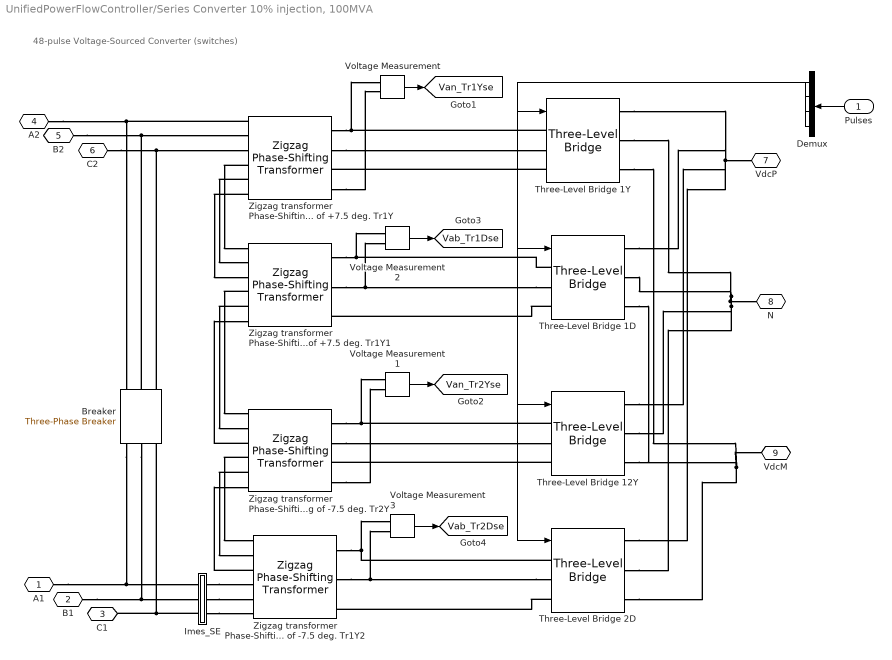
== system UnifiedPowerFlowController/Series Converter 10% injection, 100MVA ==
  note: 48-pulse Voltage-Sourced Converter
      | (switches)
  Pulses : Inport  PortDimensions=48
  Breaker : spsThreePhaseBreakerLib/Three-Phase Breaker  InitialState=closed  SwitchA=on  SwitchB=on  SwitchC=on  SwitchTimes=[ 0]  External=off  BreakerResistance=0.0001  SnubberResistance=1e6  SnubberCapacitance=inf  Measurements=None
      settings: AttributesFormatString=\n
  Demux : Demux  Outputs=[12 12 12 12]
      settings: DisplayOption=none
  Imes_SE : Subsystem
  Three-Level Bridge 12Y : spsThreeLevelBridgeLib/Three-Level Bridge  Arms=3  SnubberResistance=1e5  SbubberCapacitance=inf  Device=GTO / Diodes  Ron=1e-4  ForwardVoltages="[  0  0  ]"  Measurements=None
      settings: AttributesFormatString=\n
  Three-Level Bridge 1D : spsThreeLevelBridgeLib/Three-Level Bridge  Arms=3  SnubberResistance=1e5  SbubberCapacitance=inf  Device=GTO / Diodes  Ron=1e-4  ForwardVoltages="[  0  0  ]"  Measurements=None
      settings: AttributesFormatString=\n
  Three-Level Bridge 1Y : spsThreeLevelBridgeLib/Three-Level Bridge  Arms=3  SnubberResistance=1e5  SbubberCapacitance=inf  Device=GTO / Diodes  Ron=1e-4  ForwardVoltages="[  0  0  ]"  Measurements=None
      settings: AttributesFormatString=\n
  Three-Level Bridge 2D : spsThreeLevelBridgeLib/Three-Level Bridge  Arms=3  SnubberResistance=1e5  SbubberCapacitance=inf  Device=GTO / Diodes  Ron=1e-4  ForwardVoltages="[  0  0  ]"  Measurements=None
      settings: AttributesFormatString=\n
  Voltage Measurement{,1..3} (4 alike) : spsVoltageMeasurementLib/Voltage Measurement  Tag=PoWeRsYsTeMmEaSuReMeNt  PhasorSimulation=off  OutputType=Magnitude  PSBequivalent=0
  Zigzag transformer Phase-Shifting of +7.5 deg. Tr1Y : spsZigzagPhaseShiftingTransformerLib/Zigzag Phase-Shifting Transformer  SecondaryConnection=Yn  SetSaturation=off  SetInitialFlux=off  Measurements=None  UNITS=pu  NominalPower=[ 100e6/4 60]  PrimaryVoltage=12.5e3  SecondaryVoltage="[ 12.5e3  +7.5]"  Winding1=[ 0.05/30 0.05 ]  Winding2=[ 0.05/30 0.05 ]  Winding3=[ 0.05/30 0.05 ]  RmLm=[ 500 500 ]  Rm=500  Saturation=[ 0,0 ; 0.0024,1.2 ; 1.0,1.52 ]  InitialFluxes=[0,0,0]  BreakLoop=off  DiscreteSolver=Trapezoidal iterative  DataType=off
      settings: AttributesFormatString=\n
  Zigzag transformer Phase-Shifting of +7.5 deg. Tr1Y1 : spsZigzagPhaseShiftingTransformerLib/Zigzag Phase-Shifting Transformer  SecondaryConnection=Delta D1(-30 deg.)  SetSaturation=off  SetInitialFlux=off  Measurements=None  UNITS=pu  NominalPower=[ 100e6/4 60]  PrimaryVoltage=12.5e3  SecondaryVoltage="[ 12.5e3  +7.5]"  Winding1=[ 0.05/30 0.05 ]  Winding2=[ 0.05/30 0.05 ]  Winding3=[ 0.05/30 0.05 ]  RmLm=[ 500 500 ]  Rm=500  Saturation=[ 0,0 ; 0.0024,1.2 ; 1.0,1.52 ]  InitialFluxes=[0,0,0]  BreakLoop=off  DiscreteSolver=Trapezoidal iterative  DataType=off
      settings: AttributesFormatString=\n
  Zigzag transformer Phase-Shifting of -7.5 deg. Tr1Y2 : spsZigzagPhaseShiftingTransformerLib/Zigzag Phase-Shifting Transformer  SecondaryConnection=Delta D1(-30 deg.)  SetSaturation=off  SetInitialFlux=off  Measurements=None  UNITS=pu  NominalPower=[ 100e6/4 60]  PrimaryVoltage=12.5e3  SecondaryVoltage="[ 12.5e3  -7.5]"  Winding1=[ 0.05/30 0.05 ]  Winding2=[ 0.05/30 0.05 ]  Winding3=[ 0.05/30 0.05 ]  RmLm=[ 500 500 ]  Rm=500  Saturation=[ 0,0 ; 0.0024,1.2 ; 1.0,1.52 ]  InitialFluxes=[0,0,0]  BreakLoop=off  DiscreteSolver=Trapezoidal iterative  DataType=off
      settings: AttributesFormatString=\n
  Zigzag transformer Phase-Shifting of -7.5 deg. Tr2Y : spsZigzagPhaseShiftingTransformerLib/Zigzag Phase-Shifting Transformer  SecondaryConnection=Yn  SetSaturation=off  SetInitialFlux=off  Measurements=None  UNITS=pu  NominalPower=[ 100e6/4 60]  PrimaryVoltage=12.5e3  SecondaryVoltage="[ 12.5e3  -7.5]"  Winding1=[ 0.05/30 0.05 ]  Winding2=[ 0.05/30 0.05 ]  Winding3=[ 0.05/30 0.05 ]  RmLm=[ 500 500 ]  Rm=500  Saturation=[ 0,0 ; 0.0024,1.2 ; 1.0,1.52 ]  InitialFluxes=[0,0,0]  BreakLoop=off  DiscreteSolver=Trapezoidal iterative  DataType=off
      settings: AttributesFormatString=\n
  "A1 " : PMIOPort  Side=Left
  "B1 " : PMIOPort  Port=2  Side=Left
  C1 : PMIOPort  Port=3  Side=Left
  "A2 " : PMIOPort  Port=4  Side=Left
  "B2 " : PMIOPort  Port=5  Side=Left
  "C2 " : PMIOPort  Port=6  Side=Left
  VdcP : PMIOPort  Port=7  Side=Right
  N : PMIOPort  Port=8  Side=Right
  VdcM : PMIOPort  Port=9  Side=Right
  tag scope: Vab_Tr1Dse=global, Vab_Tr2Dse=global, Van_Tr1Yse=global, Van_Tr2Yse=global
  wires:
  Pulses/1 -> Demux/1
  Demux/4 -> Three-Level Bridge 2D/1
  Demux/3 -> Three-Level Bridge 12Y/1
  Demux/2 -> Three-Level Bridge 1D/1
  Demux/1 -> Three-Level Bridge 1Y/1
  Voltage Measurement3/1 -> [Vab_Tr2Dse]
  Voltage Measurement2/1 -> [Vab_Tr1Dse]
  Voltage Measurement1/1 -> [Van_Tr2Yse]
  Voltage Measurement/1 -> [Van_Tr1Yse]
  connections:
  Zigzag transformer Phase-Shifting of -7.5 deg. Tr2Y/RConn4 -- Voltage Measurement1/LConn2
  Zigzag transformer Phase-Shifting of +7.5 deg. Tr1Y/RConn4 -- Voltage Measurement/LConn2
  Three-Level Bridge 1Y/RConn3 -- VdcM/RConn1 -- Three-Level Bridge 1D/RConn3 -- Three-Level Bridge 2D/RConn3 -- Three-Level Bridge 12Y/RConn3
  Three-Level Bridge 12Y/RConn2 -- Three-Level Bridge 1D/RConn2 -- Three-Level Bridge 1Y/RConn2 -- N/RConn1 -- Three-Level Bridge 2D/RConn2
  Three-Level Bridge 1Y/RConn1 -- VdcP/RConn1 -- Three-Level Bridge 1D/RConn1 -- Three-Level Bridge 12Y/RConn1 -- Three-Level Bridge 2D/RConn1
  Three-Level Bridge 1D/LConn1 -- Zigzag transformer Phase-Shifting of +7.5 deg. Tr1Y1/RConn1 -- Voltage Measurement2/LConn1
  Imes_SE/RConn1 -- Zigzag transformer Phase-Shifting of -7.5 deg. Tr1Y2/LConn4
  Imes_SE/RConn2 -- Zigzag transformer Phase-Shifting of -7.5 deg. Tr1Y2/LConn5
  Imes_SE/RConn3 -- Zigzag transformer Phase-Shifting of -7.5 deg. Tr1Y2/LConn6
  "A1 "/RConn1 -- Imes_SE/LConn1 -- Breaker/RConn1
  Zigzag transformer Phase-Shifting of +7.5 deg. Tr1Y/LConn4 -- Zigzag transformer Phase-Shifting of +7.5 deg. Tr1Y1/LConn1
  Zigzag transformer Phase-Shifting of +7.5 deg. Tr1Y/LConn5 -- Zigzag transformer Phase-Shifting of +7.5 deg. Tr1Y1/LConn2
  Zigzag transformer Phase-Shifting of +7.5 deg. Tr1Y/LConn6 -- Zigzag transformer Phase-Shifting of +7.5 deg. Tr1Y1/LConn3
  Zigzag transformer Phase-Shifting of +7.5 deg. Tr1Y1/LConn4 -- Zigzag transformer Phase-Shifting of -7.5 deg. Tr2Y/LConn1
  Zigzag transformer Phase-Shifting of +7.5 deg. Tr1Y1/LConn5 -- Zigzag transformer Phase-Shifting of -7.5 deg. Tr2Y/LConn2
  Zigzag transformer Phase-Shifting of -7.5 deg. Tr2Y/LConn3 -- Zigzag transformer Phase-Shifting of +7.5 deg. Tr1Y1/LConn6
  Zigzag transformer Phase-Shifting of -7.5 deg. Tr2Y/LConn4 -- Zigzag transformer Phase-Shifting of -7.5 deg. Tr1Y2/LConn1
  Zigzag transformer Phase-Shifting of -7.5 deg. Tr2Y/LConn5 -- Zigzag transformer Phase-Shifting of -7.5 deg. Tr1Y2/LConn2
  Zigzag transformer Phase-Shifting of -7.5 deg. Tr1Y2/LConn3 -- Zigzag transformer Phase-Shifting of -7.5 deg. Tr2Y/LConn6
  Three-Level Bridge 1Y/LConn1 -- Zigzag transformer Phase-Shifting of +7.5 deg. Tr1Y/RConn1 -- Voltage Measurement/LConn1
  Three-Level Bridge 12Y/LConn1 -- Zigzag transformer Phase-Shifting of -7.5 deg. Tr2Y/RConn1 -- Voltage Measurement1/LConn1
  Three-Level Bridge 2D/LConn1 -- Zigzag transformer Phase-Shifting of -7.5 deg. Tr1Y2/RConn1 -- Voltage Measurement3/LConn1
  Imes_SE/LConn3 -- Breaker/RConn3 -- C1/RConn1
  "B1 "/RConn1 -- Imes_SE/LConn2 -- Breaker/RConn2
  Breaker/LConn3 -- Zigzag transformer Phase-Shifting of +7.5 deg. Tr1Y/LConn3 -- "C2 "/RConn1
  Breaker/LConn2 -- Zigzag transformer Phase-Shifting of +7.5 deg. Tr1Y/LConn2 -- "B2 "/RConn1
  Zigzag transformer Phase-Shifting of +7.5 deg. Tr1Y/LConn1 -- Breaker/LConn1 -- "A2 "/RConn1
  Three-Level Bridge 1Y/LConn3 -- Zigzag transformer Phase-Shifting of +7.5 deg. Tr1Y/RConn3
  Zigzag transformer Phase-Shifting of +7.5 deg. Tr1Y/RConn2 -- Three-Level Bridge 1Y/LConn2
  Three-Level Bridge 1D/LConn2 -- Zigzag transformer Phase-Shifting of +7.5 deg. Tr1Y1/RConn2 -- Voltage Measurement2/LConn2
  Three-Level Bridge 1D/LConn3 -- Zigzag transformer Phase-Shifting of +7.5 deg. Tr1Y1/RConn3
  Zigzag transformer Phase-Shifting of -7.5 deg. Tr2Y/RConn2 -- Three-Level Bridge 12Y/LConn2
  Three-Level Bridge 12Y/LConn3 -- Zigzag transformer Phase-Shifting of -7.5 deg. Tr2Y/RConn3
  Three-Level Bridge 2D/LConn2 -- Zigzag transformer Phase-Shifting of -7.5 deg. Tr1Y2/RConn2 -- Voltage Measurement3/LConn2
  Three-Level Bridge 2D/LConn3 -- Zigzag transformer Phase-Shifting of -7.5 deg. Tr1Y2/RConn3
